simulink model "comunicacion_arduno"  (R2023b)
settings: Solver=VariableStepAuto  StartTime=0.0  StopTime=inf  RelTol=1e-3
undefined symbols (not defined in the file): KD, KI, KP, LF
libraries: instrumentseriallib x3, svdutilitieslib x1
settings Model: Creator=dcasta25  LastModifiedBy=David

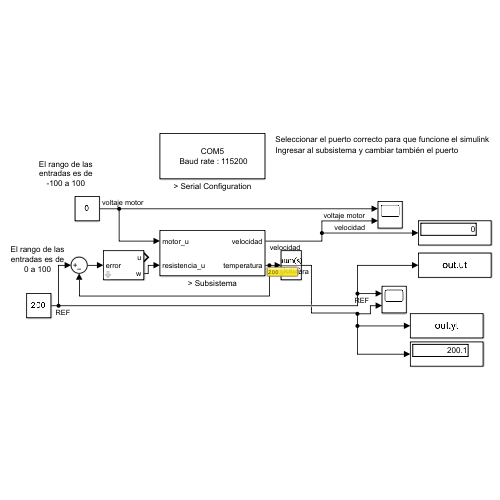
[thumbnail: Simulink's stored preview of the top-level diagram]
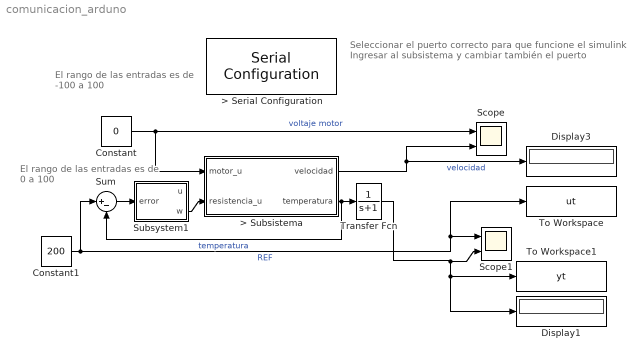
== system comunicacion_arduno ==
  note: El rango de las entradas es de 0 a 100
  note: Seleccionar el puerto correcto para que funcione el simulink
      | Ingresar al subsistema y cambiar también el puerto
  note: El rango de las entradas es de -100 a 100
  > Serial Configuration : instrumentseriallib/Serial Configuration  Priority=-200000  PortSel=COM5  Port=COM5  ComPort=COM5  BaudRate=115200  DataBits=8  Parity=none  StopBits=1  ByteOrder=little-endian  FlowControl=none  Timeout=10  SimulateUsing=Interpreted execution  BlockInModel=on  aMode=1
      settings: LibrarySourceBlock=c2000lib/Host Communication/Serial Configuration
  > Subsistema : Subsystem
      mask Display: image('$imagefile'); % Use "Edit Image" on toolstrip to change.
  Constant : Constant  Value=0
  Constant1 : Constant  Value=200
  Display1 : Display
  Display3 : Display
  Scope : Scope  NumInputPorts=2
  Scope1 : Scope  NumInputPorts=2
  Subsystem1 : Subsystem  mask{P=KP, I=KI, D=KD}
      mask prompts: P "Constante Propocional Kp"; I "Constante Integral Ki"; D "Constante Derivativa Kd"
  Sum : Sum  Inputs=|+-
  To Workspace : ToWorkspace  VariableName=ut  SaveFormat=Timeseries  SampleTime=-1
  To Workspace1 : ToWorkspace  VariableName=yt  SaveFormat=Timeseries  SampleTime=-1
  Transfer Fcn : TransferFcn  Denominator=[1 1]
  wires:
  > Subsistema/1(velocidad) -> Display3/1, Scope/2  "velocidad"
  Constant/1 -> > Subsistema/1(motor_u), Scope/1  "voltaje motor"
  Constant1/1 -> To Workspace/1, Scope1/1, Sum/1  "REF"
  > Subsistema/2(temperatura) -> Sum/2, Transfer Fcn/1  "temperatura"
  Subsystem1/2(w) -> > Subsistema/2(resistencia_u)
  Sum/1 -> Subsystem1/1(error)
  Transfer Fcn/1 -> Display1/1, To Workspace1/1, Scope1/2

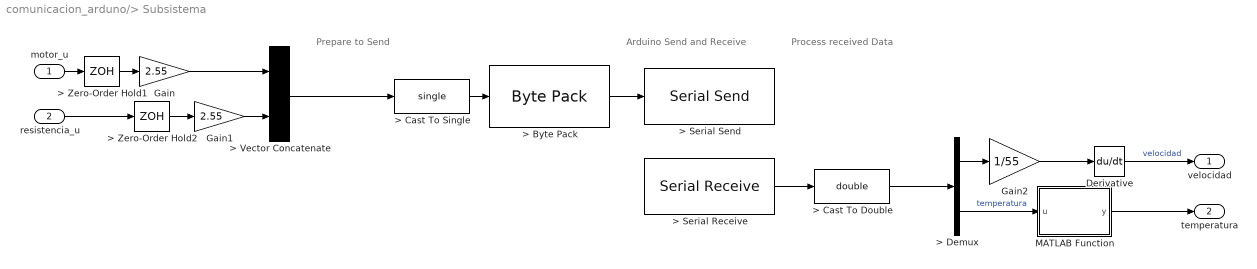
== system comunicacion_arduno/> Subsistema ==
  note: Process received Data
  note: Arduino Send and Receive
  note: Prepare to Send
  motor_u : Inport
  resistencia_u : Inport  Port=2
  > Byte Pack : svdutilitieslib/Byte Pack  maskPackedDataType=uint32  datatypes={'single'}  byteAlign=4  blockPlatform=tic2000
      settings: LibrarySourceBlock=c2000lib/Target Communication/Byte Pack
  > Cast To Double : DataTypeConversion  OutDataTypeStr=double  SaturateOnIntegerOverflow=off  RndMeth=Floor
  > Cast To Single : DataTypeConversion  OutDataTypeStr=single  SaturateOnIntegerOverflow=off  RndMeth=Floor
  > Demux : Demux  Outputs=2
  > Serial Receive : instrumentseriallib/Serial Receive  Priority=1  PortSel=COM5  Port=COM5  ComPort=COM5  DataType=single  SaveDataType=uint8  ToggleHeader=on  Header=uint8('A')  ToggleTerminator=on  Terminator=LF ('\n')  CustomTerminator=[]  InputFormat=Column major  ToggleDataSize=on  DataSize=[1 2]  EnableBlockingMode=on  ActionDataUnavailable=Output last received value  ActionWhenDataUnavailable=Output last received value  CustomValue=0  SampleTime=0.05  SimulateUsing=Interpreted execution  BlockInModel=on  aMode=1
      settings: LibrarySourceBlock=c2000lib/Host Communication/Serial Receive
  > Serial Send : instrumentseriallib/Serial Send  Priority=1  PortSel=COM5  Port=COM5  ComPort=COM5  Header=[]  Terminator=<none>  CustomTerminator=[]  EnableBlockingMode=on  SimulateUsing=Interpreted execution  BlockInModel=on  aMode=1
      settings: LibrarySourceBlock=c2000lib/Host Communication/Serial Send
  > Vector Concatenate : Concatenate
  > Zero-Order Hold1 : ZeroOrderHold  SampleTime=0.05
  > Zero-Order Hold2 : ZeroOrderHold  SampleTime=0.05
  Derivative : Derivative
  Gain : Gain  Gain=2.55
  Gain1 : Gain  Gain=2.55
  Gain2 : Gain  Gain=1/55
  MATLAB Function : MATLAB Function  TreatAsAtomicUnit=on
  velocidad : Outport
  temperatura : Outport  Port=2
  wires:
  > Vector Concatenate/1 -> > Cast To Single/1
  > Cast To Single/1 -> > Byte Pack/1
  > Cast To Double/1 -> > Demux/1
  > Byte Pack/1 -> > Serial Send/1
  resistencia_u/1 -> > Zero-Order Hold2/1
  Derivative/1 -> velocidad/1  "velocidad"
  > Serial Receive/1 -> > Cast To Double/1
  > Demux/1 -> Gain2/1
  > Demux/2 -> MATLAB Function/1(u)  "temperatura"
  motor_u/1 -> > Zero-Order Hold1/1
  Gain/1 -> > Vector Concatenate/1
  Gain1/1 -> > Vector Concatenate/2
  > Zero-Order Hold1/1 -> Gain/1
  > Zero-Order Hold2/1 -> Gain1/1
  Gain2/1 -> Derivative/1
  MATLAB Function/1(y) -> temperatura/1

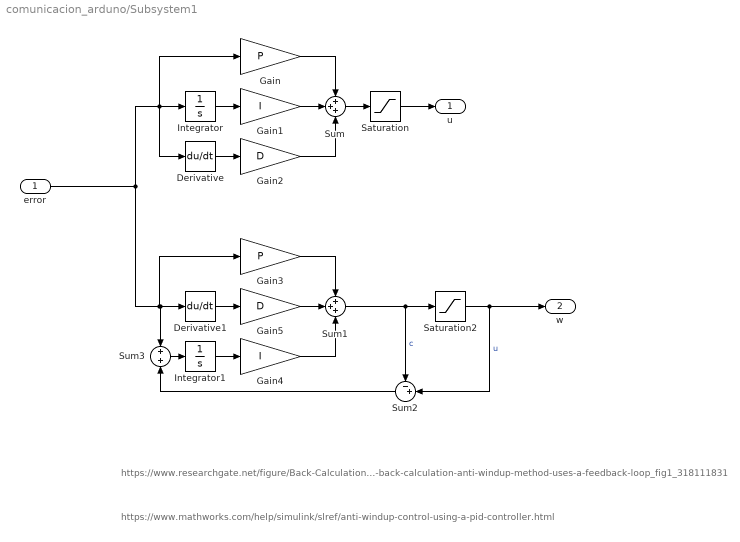
== system comunicacion_arduno/Subsystem1 ==
  note: https://www.mathworks.com/help/simulink/slref/anti-windup-control-using-a-pid-controller.html
  note: https://www.researchgate.net/figure/Back-Calculation-algorithm-The-back-calculation-anti-windup-method-uses-a-feedback-loop_fig1_318111831
  error : Inport
  Derivative : Derivative
  Derivative1 : Derivative
  Gain : Gain  Gain=P
  Gain1 : Gain  Gain=I
  Gain2 : Gain  Gain=D
  Gain3 : Gain  Gain=P
  Gain4 : Gain  Gain=I
  Gain5 : Gain  Gain=D
  Integrator : Integrator
  Integrator1 : Integrator
  Saturation : Saturate  UpperLimit=100  LowerLimit=0
  Saturation2 : Saturate  UpperLimit=100  LowerLimit=0
  Sum : Sum  Inputs=+++
  Sum1 : Sum  Inputs=+++
  Sum2 : Sum  Inputs=-+|
  Sum3 : Sum  Inputs=+|+
  u : Outport
  w : Outport  Port=2
  wires:
  Derivative/1 -> Gain2/1
  Integrator/1 -> Gain1/1
  Gain1/1 -> Sum/2
  Gain/1 -> Sum/1
  Gain2/1 -> Sum/3
  Sum/1 -> Saturation/1
  Saturation/1 -> u/1
  Integrator1/1 -> Gain4/1
  Gain3/1 -> Sum1/1
  Derivative1/1 -> Gain5/1
  error/1 -> Sum3/1, Derivative1/1, Gain3/1, Derivative/1, Gain/1, Integrator/1
  Sum1/1 -> Saturation2/1, Sum2/1  "c"
  Saturation2/1 -> w/1, Sum2/2  "u"
  Gain5/1 -> Sum1/2
  Gain4/1 -> Sum1/3
  Sum3/1 -> Integrator1/1
  Sum2/1 -> Sum3/2

== matlab function comunicacion_arduno/> Subsistema/MATLAB Function ==
  data: u input; y output
function y = fcn(u)

RA = 220;
PA=0.00126890587593187;
PB=0.000109535819898085;
PC=6.21765891580107E-07;
Kelvin = 273.15;

R = RA*(1023/u-1);
y = 1/(PA+PB*log(R)+PC*log(R)^3)-Kelvin;
